simulink model "e5_Quadrotor_3_blocks"  (R2020a)
settings: Solver=FixedStepAuto  StartTime=0.0  StopTime=options.T_train  FixedStep=options.dt  RelTol=1e-6
undefined symbols (not defined in the file or in its folder): options, Quad
libraries: neural x69, simulink x3
(part 6 of 6)

== system e5_Quadrotor_3_blocks/NN/Layer 3/Delays 1 ==
  "p{3}" : Inport  PortDimensions=30
      mask Display: e = 0.06;c1 = [120 230 180]/255;c2 = ([120 230 180]+0)/(256+128);c3 = ([120 230 180]+128)/(256+128);patch([0 1 1 0],[0 0 1 1],c1);patch([0 1 1 1-e 1-e 0+e],[0 0 1 1-e 0+e 0+e],c2);patch([0 0 1 1-e 0+e 0+e],[0 1 1 1-e 1-e 0+e],c3);plot([0 1 1 0 0],[0 0 1 1 0]);
  mux : Mux  Inputs=1
      mask Display: e = 0.06;c1 = [120 150 230]/255;c2 = ([120 150 230]+0)/383;c3 = ([120 150 230]+128)/383;patch([0 1 1 0],[0 0 1 1],c1);patch([0 1 1 1-e 1-e 0+e],[0 0 1 1-e 0+e 0+e],c2);patch([0 0 1 1-e 0+e 0+e],[0 1 1 1-e 1-e 0+e],c3);plot([0 1 1 0 0],[0 0 1 1 0]);disp('Mux')
  "pd{3,2}" : Outport
      mask Display: e = 0.06;c1 = [120 230 180]/255;c2 = ([120 230 180]+0)/(256+128);c3 = ([120 230 180]+128)/(256+128);patch([0 1 1 0],[0 0 1 1],c1);patch([0 1 1 1-e 1-e 0+e],[0 0 1 1-e 0+e 0+e],c2);patch([0 0 1 1-e 0+e 0+e],[0 1 1 1-e 1-e 0+e],c3);plot([0 1 1 0 0],[0 0 1 1 0]);
  wires:
  "p{3}"/1 -> mux/1
  mux/1 -> "pd{3,2}"/1

== system e5_Quadrotor_3_blocks/NN/Layer 3/LW{3,2} ==
  "ad{3,2}" : Inport  PortDimensions=30
      mask Display: e = 0.06;c1 = [120 230 180]/255;c2 = ([120 230 180]+0)/(256+128);c3 = ([120 230 180]+128)/(256+128);patch([0 1 1 0],[0 0 1 1],c1);patch([0 1 1 1-e 1-e 0+e],[0 0 1 1-e 0+e 0+e],c2);patch([0 0 1 1-e 0+e 0+e],[0 1 1 1-e 1-e 0+e],c3);plot([0 1 1 0 0],[0 0 1 1 0]);
  "IW{3,2}(1,:)'" : Constant  Value=[-0.51254678109572238131619315026910044252872467041015625;-0.2303909649563717076947710893364273943006992340087890625;0.95221744076471626083701949028181843459606170654296875;0.13562594515480075330060572014190256595611572265625;0.432760096545067918238913762252195738255977630615234375;-0.65785664024319989717781709259725175797939300537109375;-0.80431495918778328491072215911117382347583770751953125;-0.467216613185155171805718055111356079578399658203125;0.85756622485518663179249188033281825482845306396484375;-1.079570188496807414679778958088718354701995849609375;1.409678490260338978856680114404298365116119384765625;0.2357383511978932144614873323007486760616302490234375;-0.2221620960290356661115396263994625769555568695068359375;-1.0404642368171364008588852811953984200954437255859375;0.1339108716278248623066104983081459067761898040771484375;0.19329795122655990535776027172687463462352752685546875;-1.07826169315540720816670727799646556377410888671875;0.5161368103069390311787856262526474893093109130859375;0.2151014170117664381365329973050393164157867431640625;0.1773628602912949714376367182921967469155788421630859375;-0.33735184994066003127954900264739990234375;0.48424888905151652895852976143942214548587799072265625;0.71903514644836530322891121613793075084686279296875;-0.485846177137463641759751453719218261539936065673828125;0.85327232575430167482721799387945793569087982177734375;-0.587372813762468748421952113858424127101898193359375;0.55534309923542224396442179568111896514892578125;0.1700725875899853634098946031372179277241230010986328125;-0.11710187423212549406859039891060092486441135406494140625;-0.52074978387466985818576858946471475064754486083984375]
      mask Display: e = 0.06;c1 = [120 150 230]/255;c2 = ([120 150 230]+0)/383;c3 = ([120 150 230]+128)/383;patch([0 1 1 0],[0 0 1 1],c1);patch([0 1 1 1-e 1-e 0+e],[0 0 1 1-e 0+e 0+e],c2);patch([0 0 1 1-e 0+e 0+e],[0 1 1 1-e 1-e 0+e],c3);plot([0 1 1 0 0],[0 0 1 1 0]);disp('weights');
  "IW{3,2}(2,:)'" : Constant  Value=[0.0167868277112131203399059131697867996990680694580078125;0.6433025990084189071893661093781702220439910888671875;-0.0249062619432176314548943452109597274102270603179931640625;0.741166906855656559827139062690548598766326904296875;0.84120628472185654533888055084389634430408477783203125;0.00292163504752237894457334022035865928046405315399169921875;-0.322235864613730271788227810247917659580707550048828125;0.55757722486574967657446677549160085618495941162109375;-0.060061794741713740719557534930572728626430034637451171875;-0.0751090708586184818695841158842085860669612884521484375;0.1715472210139683817420319655866478569805622100830078125;0.308407261725961057141631727063213475048542022705078125;-0.25494728719327552912687906427890993654727935791015625;0.0160178023944187557237039953861312824301421642303466796875;0.220012929405573043339927608030848205089569091796875;0.58233650721528251725800373606034554541110992431640625;0.12485951865100496094296289584235637448728084564208984375;-0.5985825527929076184108225788804702460765838623046875;0.70267029025257976559970529706333763897418975830078125;0.1178911029522342612807506156968884170055389404296875;-0.0249335182470433215640159829717958928085863590240478515625;0.2203484064432011113598974816341069526970386505126953125;-0.160112198699139229862709044027724303305149078369140625;-0.2106381170686273673897659364229184575378894805908203125;-0.3572785580075914513287216323078610002994537353515625;-0.1388136228256115212165155980983399786055088043212890625;-0.383056897240806659699074998570722527801990509033203125;0.72829414672149483944707526461570523679256439208984375;0.158142951744333071228965081900241784751415252685546875;0.5880812307672282912562877754680812358856201171875]
      mask Display: e = 0.06;c1 = [120 150 230]/255;c2 = ([120 150 230]+0)/383;c3 = ([120 150 230]+128)/383;patch([0 1 1 0],[0 0 1 1],c1);patch([0 1 1 1-e 1-e 0+e],[0 0 1 1-e 0+e 0+e],c2);patch([0 0 1 1-e 0+e 0+e],[0 1 1 1-e 1-e 0+e],c3);plot([0 1 1 0 0],[0 0 1 1 0]);disp('weights');
  "IW{3,2}(3,:)'" : Constant  Value=[0.0112564591745442331427451421177465817891061305999755859375;-0.7079537681103731383558397283195517957210540771484375;-0.28389312629468987925207557054818607866764068603515625;0.147572667946573476971394711654284037649631500244140625;1.005811525046080401324388731154613196849822998046875;0.07203680127190602300313315708990558050572872161865234375;-0.56661575765124094772318130708299577236175537109375;0.4100090694083002862413422917597927153110504150390625;0.044486614628830432882633516555870301090180873870849609375;-0.31737417493607844587444333228631876409053802490234375;0.092431042782106287436505454024882055819034576416015625;-0.56764791244586643159664163249544799327850341796875;-0.08955862280071315295604250650285393930971622467041015625;0.0569163630811010679000361278667696751654148101806640625;-0.126735890443810228500609582624747417867183685302734375;-0.442743957720037162317794354748912155628204345703125;-0.021786826540171590205208218549159937538206577301025390625;0.293161019711157322387151680231909267604351043701171875;-0.8747457268957046228052831793320365250110626220703125;0.1821254313549623138346333917070296593010425567626953125;-0.534309044116886067143923355615697801113128662109375;0.2925319830870016790669296824489720165729522705078125;0.0310008261521734045096376775063617969863116741180419921875;0.10085519270528464641500931975315324962139129638671875;-0.341727378836315820453961578095913864672183990478515625;-0.25649797410892094529089035859215073287487030029296875;0.08888951895600684383058620596784749068319797515869140625;-0.86924217289554572829501921660266816616058349609375;0.6758635281012370654707410722039639949798583984375;-0.296376809561871457088244596889126114547252655029296875]
      mask Display: e = 0.06;c1 = [120 150 230]/255;c2 = ([120 150 230]+0)/383;c3 = ([120 150 230]+128)/383;patch([0 1 1 0],[0 0 1 1],c1);patch([0 1 1 1-e 1-e 0+e],[0 0 1 1-e 0+e 0+e],c2);patch([0 0 1 1-e 0+e 0+e],[0 1 1 1-e 1-e 0+e],c3);plot([0 1 1 0 0],[0 0 1 1 0]);disp('weights');
  "IW{3,2}(4,:)'" : Constant  Value=[0.6125087988180950571148741801152937114238739013671875;-0.60694407614783718596385142518556676805019378662109375;0.91900487801871200144177009860868565738201141357421875;0.6143561433623461187636394242872484028339385986328125;-0.1822798840945272502711560491661657579243183135986328125;0.04479238415941437512213241234348970465362071990966796875;-0.308732719858687387759488274241448380053043365478515625;-0.517802265967414410141600455972366034984588623046875;-0.2156047990574780082173589335070573724806308746337890625;0.536083438599389783263404751778580248355865478515625;-0.259572781841144628600659416406415402889251708984375;0.27413821588714315513612973518320359289646148681640625;-0.61927889574570638142603229425731115043163299560546875;0.07955739547322117355410142636173986829817295074462890625;0.71649303718654666628395943916984833776950836181640625;0.43961588650559269009221452506608329713344573974609375;0.468556491531269270200965593176078982651233673095703125;0.47081338847110743017765344120562076568603515625;-0.61057044440077790081744524286477826535701751708984375;-0.871842340848128838359798464807681739330291748046875;-0.696120732527408581091776795801706612110137939453125;0.352021237036145573373602246647351421415805816650390625;-0.406674343162727602862815956541453488171100616455078125;-0.789234022852547401072342836414463818073272705078125;0.3585775622641858007000337238423526287078857421875;-0.3359283034298738979117615599534474313259124755859375;-1.052636110354225440488562526297755539417266845703125;0.6702062746552697181101621026755310595035552978515625;0.2091478727148194660667712696522357873618602752685546875;0.11428141370061284387560363029479049146175384521484375]
      mask Display: e = 0.06;c1 = [120 150 230]/255;c2 = ([120 150 230]+0)/383;c3 = ([120 150 230]+128)/383;patch([0 1 1 0],[0 0 1 1],c1);patch([0 1 1 1-e 1-e 0+e],[0 0 1 1-e 0+e 0+e],c2);patch([0 0 1 1-e 0+e 0+e],[0 1 1 1-e 1-e 0+e],c3);plot([0 1 1 0 0],[0 0 1 1 0]);disp('weights');
  Mux : Mux
      mask Display: e = 0.06;c1 = [120 150 230]/255;c2 = ([120 150 230]+0)/383;c3 = ([120 150 230]+128)/383;patch([0 1 1 0],[0 0 1 1],c1);patch([0 1 1 1-e 1-e 0+e],[0 0 1 1-e 0+e 0+e],c2);patch([0 0 1 1-e 0+e 0+e],[0 1 1 1-e 1-e 0+e],c3);plot([0 1 1 0 0],[0 0 1 1 0]);disp('Mux');
  dotprod{1..4} (4 alike) : neural/Weight Functions/dotprod
  "lz{3,2}" : Outport
      mask Display: e = 0.06;c1 = [120 230 180]/255;c2 = ([120 230 180]+0)/(256+128);c3 = ([120 230 180]+128)/(256+128);patch([0 1 1 0],[0 0 1 1],c1);patch([0 1 1 1-e 1-e 0+e],[0 0 1 1-e 0+e 0+e],c2);patch([0 0 1 1-e 0+e 0+e],[0 1 1 1-e 1-e 0+e],c3);plot([0 1 1 0 0],[0 0 1 1 0]);
  wires:
  "IW{3,2}(1,:)'"/1 -> dotprod1/1
  "ad{3,2}"/1 -> dotprod1/2, dotprod2/2, dotprod3/2, dotprod4/2
  dotprod1/1 -> Mux/1
  "IW{3,2}(2,:)'"/1 -> dotprod2/1
  dotprod2/1 -> Mux/2
  "IW{3,2}(3,:)'"/1 -> dotprod3/1
  dotprod3/1 -> Mux/3
  "IW{3,2}(4,:)'"/1 -> dotprod4/1
  dotprod4/1 -> Mux/4
  Mux/1 -> "lz{3,2}"/1
